simulink model "Lab1PartA2"  (R2016a)
settings: Solver=VariableStepAuto  StartTime=0.0  StopTime=20.0  RelTol=1e-3
settings Model: Creator=pzastawn  LastModifiedBy=pzastawn

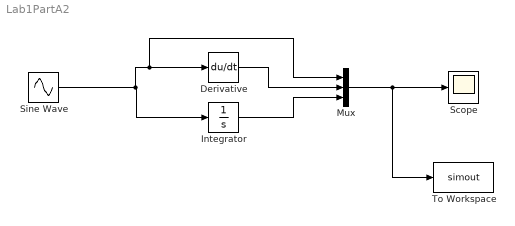
== system Lab1PartA2 ==
  Derivative : Derivative
  Integrator : Integrator
  Mux : Mux  Inputs=3
  Scope : Scope
  Sine Wave : Sin  Frequency=1.257  SampleTime=0
  To Workspace : ToWorkspace  VariableName=simout  SaveFormat=Timeseries  SampleTime=-1
  wires:
  Sine Wave/1 -> Mux/1, Derivative/1, Integrator/1
  Mux/1 -> To Workspace/1, Scope/1
  Derivative/1 -> Mux/2
  Integrator/1 -> Mux/3
